simulink model "TCLab_Test_PIL"  (R2026a)
settings: Solver=FixedStepDiscrete  StopTime=t_final  FixedStep=Ts  EnableMultiTasking=on
InitFcn:
  | init_TCLab_SIMC
values from neighbouring files (symbols this model uses):
  den_Gp_d = [1 -0.994731114001]    [ELWORKSPACE.mat]
  num_Gp_d = [0 0.00494116655898]    [ELWORKSPACE.mat]
  T_amb = 25    [A8_init_TCLab_SIMC.m]    (also in ELWORKSPACE.mat; SIMC_controller_TCLab.m; init_TCLab_SIMC.m)
  T_ref = 60    [A8_init_TCLab_SIMC.m]    (also in ELWORKSPACE.mat; SIMC_controller_TCLab.m = str2double(strrep(entrada, ',', '.')); init_TCLab_SIMC.m)
  theta = 22.021    [A8_init_TCLab_SIMC.m]    (also in ELWORKSPACE.mat = 21; SIMC_controller_TCLab.m = 21; identificar_FOPDT_TCLab.m = mejorTheta; init_TCLab_SIMC.m = 21)
  Ts = 1    [A8_init_TCLab_SIMC.m]    (also in ELWORKSPACE.mat; SIMC_controller_TCLab.m; experimento_escalon_Q1_TCLab.m; experimento_multinivel_Q1_TCLab.m)
undefined symbols (not defined in the file or in its folder): dspblkCoreblockFVToolHelper, gcbh
settings Model: SimulationMode=external  SILPILSystemUnderTest=refmodels  Creator=jguerrero  LastModifiedBy=pablo
settings DebuggingCC: UnderspecifiedInitializationDetection=Classic
settings HardwareCC: ProdBitPerInt=16.0  ProdBitPerPointer=16.0  ProdBitPerSizeT=16.0  ProdBitPerPtrDiffT=16.0  ProdWordSize=8.0  ProdHWDeviceType=Atmel->AVR
settings ModelReferenceCC: PropagateVarSize=During execution
settings RTWCC: SystemTargetFile=ert.tlc  HardwareBoard=Arduino Uno  TLCOptions=-aInlineSetEventsForThisBaseRateFcn=TLC_FALSE -aSuppressMultiTaskScheduler=TLC_FALSE -aRateBasedStepFcn=1  Toolchain=Arduino AVR  BuildConfiguration=Faster Runs  PortableWordSizes=on  Description=Embedded Coder
settings ERTTargetCC: ExtModeTransport=3.0  ExtModeAutomaticAllocSize=off  ExtModeStaticAllocSize=250.0  CodeInterfacePackaging=Reusable function  SupportContinuousTime=on  SupportVariableSizeSignals=on

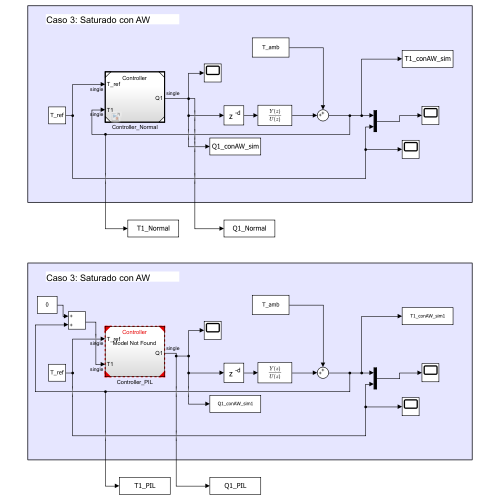
[thumbnail: Simulink's stored preview of the top-level diagram]
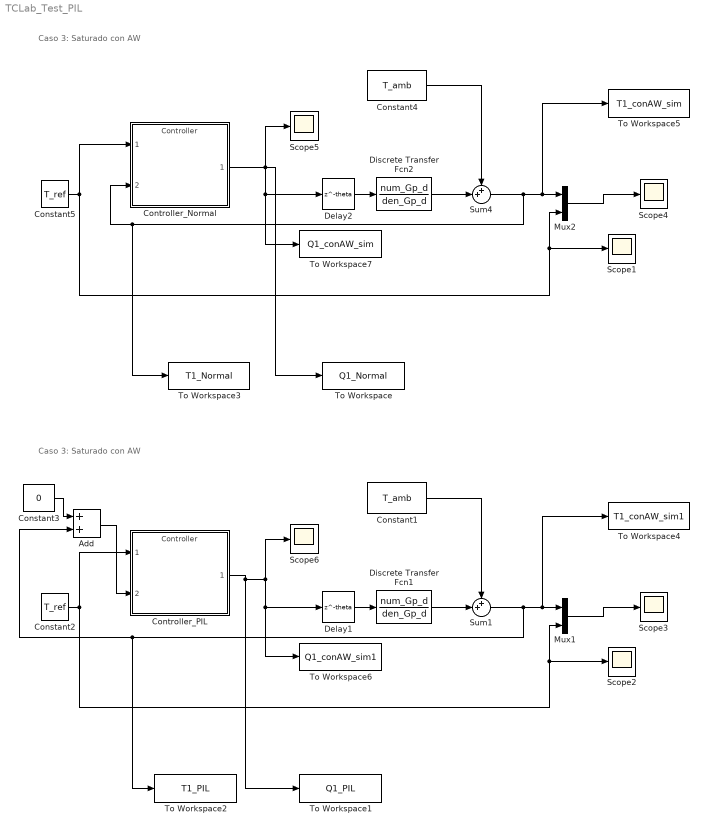
== system TCLab_Test_PIL ==
  note: Caso 3: Saturado con AW
  note: Caso 3: Saturado con AW
  Add : Sum
  Constant1 : Constant  Value=T_amb  OutDataTypeStr=single  SampleTime=Ts
  Constant2 : Constant  Value=T_ref  OutDataTypeStr=single  SampleTime=Ts
  Constant3 : Constant  Value=0  OutDataTypeStr=single  SampleTime=Ts
  Constant4 : Constant  Value=T_amb  OutDataTypeStr=single  SampleTime=Ts
  Constant5 : Constant  Value=T_ref  OutDataTypeStr=single  SampleTime=Ts
  Controller_Normal : ModelReference  ModelNameDialog=Controller  SimulationMode=Normal  ModelReferenceVersion=1.27
  Controller_PIL : ModelReference  InitFcn=init_TCLab_SIMC  ModelNameDialog=Controller  SimulationMode=Processor-in-the-loop (PIL)  ModelReferenceVersion=1.27
  Delay1 : Delay  DelayLength=theta  SampleTime=Ts
  Delay2 : Delay  DelayLength=theta  SampleTime=Ts
  Discrete Transfer Fcn1 : DiscreteTransferFcn  LoadFcn=dspblkCoreblockFVToolHelper(gcbh,'load');  Numerator=num_Gp_d  Denominator=den_Gp_d
      settings: CopyFcn=dspblkCoreblockFVToolHelper(gcbh,'copy');  DeleteFcn=dspblkCoreblockFVToolHelper(gcbh,'close');  ModelCloseFcn=dspblkCoreblockFVToolHelper(gcbh,'close');  PreSaveFcn=dspblkCoreblockFVToolHelper(gcbh,'presave');  PostSaveFcn=dspblkCoreblockFVToolHelper(gcbh,'postsave');  CloseFcn=dspblkCoreblockFVToolHelper(gcbh,'close');
  Discrete Transfer Fcn2 : DiscreteTransferFcn  LoadFcn=dspblkCoreblockFVToolHelper(gcbh,'load');  Numerator=num_Gp_d  Denominator=den_Gp_d
      settings: CopyFcn=dspblkCoreblockFVToolHelper(gcbh,'copy');  DeleteFcn=dspblkCoreblockFVToolHelper(gcbh,'close');  ModelCloseFcn=dspblkCoreblockFVToolHelper(gcbh,'close');  PreSaveFcn=dspblkCoreblockFVToolHelper(gcbh,'presave');  PostSaveFcn=dspblkCoreblockFVToolHelper(gcbh,'postsave');  CloseFcn=dspblkCoreblockFVToolHelper(gcbh,'close');
  Mux1 : Mux  Inputs=2
  Mux2 : Mux  Inputs=2
  Scope{1..6} (6 alike) : Scope
      Scope1 settings: ActiveDisplayYMinimum=49.277320799059929  ActiveDisplayYMaximum=62.429494712103406
      Scope2 settings: ActiveDisplayYMinimum=49.277320799059929  ActiveDisplayYMaximum=62.429494712103406
      Scope3 settings: ActiveDisplayYMinimum=10.038288910910744  ActiveDisplayYMaximum=60.148433319164823  DataLoggingVariableName=ScopeData2
      Scope4 settings: ActiveDisplayYMinimum=10.038288910910744  ActiveDisplayYMaximum=60.148433319164823  DataLoggingVariableName=ScopeData4
      Scope5 settings: ActiveDisplayYMinimum=30.736520647506694  ActiveDisplayYMaximum=96.58483103916592  DataLoggingVariableName=ScopeData5
      Scope6 settings: ActiveDisplayYMinimum=30.736520647506694  ActiveDisplayYMaximum=96.58483103916592  DataLoggingVariableName=ScopeData3
  Sum1 : Sum  Inputs=++|
  Sum4 : Sum  Inputs=++|
  To Workspace : ToWorkspace  VariableName=Q1_Normal  SaveFormat=Timeseries  SampleTime=1
  To Workspace1 : ToWorkspace  VariableName=Q1_PIL  SaveFormat=Timeseries  SampleTime=1
  To Workspace2 : ToWorkspace  VariableName=T1_PIL  SaveFormat=Timeseries  SampleTime=1
  To Workspace3 : ToWorkspace  VariableName=T1_Normal  SaveFormat=Timeseries  SampleTime=1
  To Workspace4 : ToWorkspace  VariableName=T1_conAW_sim1  SaveFormat=Timeseries  SampleTime=-1
  To Workspace5 : ToWorkspace  VariableName=T1_conAW_sim  SaveFormat=Timeseries  SampleTime=-1
  To Workspace6 : ToWorkspace  VariableName=Q1_conAW_sim1  SaveFormat=Timeseries  SampleTime=-1
  To Workspace7 : ToWorkspace  VariableName=Q1_conAW_sim  SaveFormat=Timeseries  SampleTime=-1
  wires:
  Constant4/1 -> Sum4/1
  Sum4/1 -> To Workspace3/1, Controller_Normal/2, Mux2/1, To Workspace5/1
  Delay2/1 -> Discrete Transfer Fcn2/1
  Discrete Transfer Fcn2/1 -> Sum4/2
  Mux2/1 -> Scope4/1
  Constant5/1 -> Controller_Normal/1, Scope1/1, Mux2/2
  Controller_Normal/1 -> To Workspace/1, To Workspace7/1, Delay2/1, Scope5/1
  Sum1/1 -> To Workspace2/1, Add/2, Mux1/1, To Workspace4/1
  Constant1/1 -> Sum1/1
  Discrete Transfer Fcn1/1 -> Sum1/2
  Controller_PIL/1 -> To Workspace1/1, To Workspace6/1, Delay1/1, Scope6/1
  Mux1/1 -> Scope3/1
  Constant2/1 -> Controller_PIL/1, Scope2/1, Mux1/2
  Delay1/1 -> Discrete Transfer Fcn1/1
  Add/1 -> Controller_PIL/2
  Constant3/1 -> Add/1
